simulink model "state_space_delay"  (R2018b)
settings: Solver=VariableStepAuto  StartTime=0.0  StopTime=5  RelTol=1e-3
values from neighbouring files (symbols this model uses):
  C = K * (k_p + 2 * s)/(1 + s/100) * (s^2 + s + 4)/(1 + s * T)^2    [continous_controller.m]    (also in disturbance_rejection.m = 20 * (10 + 2 * s + 10/s)/(1 + s/100) * (s^2 + s + 4)/(1 + s ; lqr_delay.m = eye(4); pole_placement_delay.m = eye(4))
  K_delay = place(sys_discrete.A, sys_discrete.B, discrete_poles)    [pole_placement_delay.m]
  k_r = k_r(1)^-1    [discrete_pole_placement.m]    (also in lqr_delay.m = 30)
  selector = [0, 0, 0, 1]    [lqr_delay.m]    (also in pole_placement_delay.m)
  sys_discrete = c2d(sys, 2*pi/sampling_freq, 'zoh')    [control_input_bound.m]    (also in delayed_input.m = (c2d(sys, 2*pi/sampling_freq, 'zoh')); discrete_pole_placement.m = (c2d(sys, 2*pi/sampling_freq, 'zoh')); discretization.m; lqr_controller.m)
settings Model: Creator=lorenzoterenzi  LastModifiedBy=lorenzoterenzi

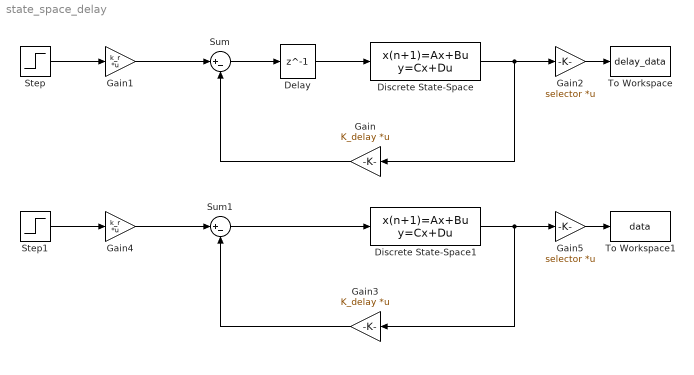
== system state_space_delay ==
  Delay : Delay  DelayLength=1  InitialCondition=0
  Discrete State-Space : DiscreteStateSpace  A=sys_discrete.A  B=sys_discrete.B  C=C  D=[0;0;0;0]  SampleTime=sys_discrete.Ts
  Discrete State-Space1 : DiscreteStateSpace  A=sys_discrete.A  B=sys_discrete.B  C=C  D=[0;0;0;0]  SampleTime=sys_discrete.Ts
  Gain : Gain  Gain=K_delay  Multiplication=Matrix(K*u)
  Gain1 : Gain  Gain=k_r  Multiplication=Matrix(K*u)
  Gain2 : Gain  Gain=selector  Multiplication=Matrix(K*u)
  Gain3 : Gain  Gain=K_delay  Multiplication=Matrix(K*u)
  Gain4 : Gain  Gain=k_r  Multiplication=Matrix(K*u)
  Gain5 : Gain  Gain=selector  Multiplication=Matrix(K*u)
  Step : Step  Time=0  SampleTime=0
  Step1 : Step  Time=0  SampleTime=0
  Sum : Sum  Inputs=|+-
  Sum1 : Sum  Inputs=|+-
  To Workspace : ToWorkspace  VariableName=delay_data  SaveFormat=Timeseries  SampleTime=-1
  To Workspace1 : ToWorkspace  VariableName=data  SaveFormat=Timeseries  SampleTime=-1
  wires:
  Gain2/1 -> To Workspace/1
  Gain/1 -> Sum/2
  Sum/1 -> Delay/1
  Discrete State-Space/1 -> Gain2/1, Gain/1
  Delay/1 -> Discrete State-Space/1
  Step/1 -> Gain1/1
  Gain1/1 -> Sum/1
  Step1/1 -> Gain4/1
  Sum1/1 -> Discrete State-Space1/1
  Gain4/1 -> Sum1/1
  Discrete State-Space1/1 -> Gain5/1, Gain3/1
  Gain5/1 -> To Workspace1/1
  Gain3/1 -> Sum1/2
